simulink model "rre"  (Simulink 7.6)
settings: Solver=ode45  SolverMode=SingleTasking  StartTime=0  StopTime=10  FixedStep=0.002  RelTol=1e-3  AbsTol=1e-6
libraries: Solver_SF x1
settings Model: Creator=ywata  LastModifiedBy=bduprey  ExtModeTrigMode=oneshot  ExtModeArmWhenConnect=off
settings DataIOCC: LimitDataPoints=off  SignalLoggingName=sigsOut
settings OptimizationCC: BlockReduction=off  BooleanDataType=off  ExpressionDepthLimit=128
settings DebuggingCC: SaveWithParameterizedLinksMsg=none  SignalResolutionControl=TryResolveAllWithWarning  SolverPrmCheckMsg=none  MultiTaskDSMMsg=warning  MultiTaskCondExecSysMsg=none  FcnCallInpInsideContextMsg=Enable All
settings HardwareCC: TargetUnknown=on
settings RTWCC: TemplateMakefile=grt_vc.tmf
settings CodeAppCC: CustomSymbolStrType=$N$R$M_T
settings GRTTargetCC: TargetFcnLib=ansi_tfl_tmw.mat  TargetFunctionLibrary=C89/C90 (ANSI)

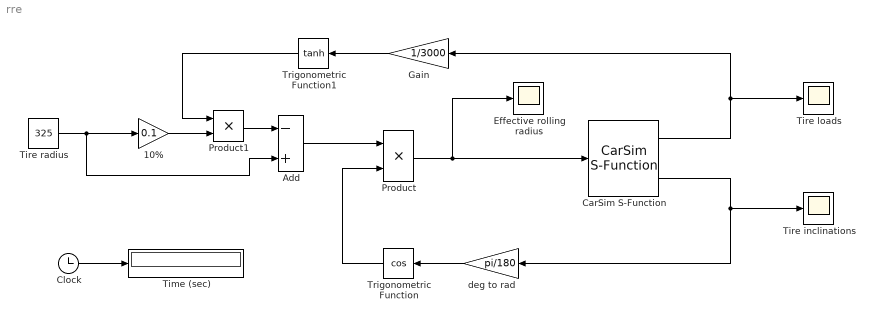
== system rre ==
  10% : Gain  Gain=0.1
  Add : Sum  Inputs=-+
  CarSim S-Function : Solver_SF/CarSim S-Function  Priority=1  SIMFILE=simfile.sim
  Clock : Clock
      settings: Decimation=10
  Effective rolling radius : Scope
      settings: TimeRange=6.3125  YMin=290  YMax=320  DataFormat=Array
  Gain : Gain  Gain=1/3000
  Product : Product
  Product1 : Product
  Time (sec) : Display
      settings: Format=bank  Decimation=100
  Tire inclinations : Scope
      settings: TimeRange=6.3125  YMin=-3  YMax=2  DataFormat=Array
  Tire loads : Scope
      settings: TimeRange=6.3125  YMin=0  YMax=6000  SaveName=ScopeData2  DataFormat=Array
  Tire radius : Constant  Value=325
  Trigonometric Function : Trigonometry  Operator=cos
  Trigonometric Function1 : Trigonometry  Operator=tanh
  deg to rad : Gain  Gain=pi/180
  wires:
  Clock/1 -> Time (sec)/1
  deg to rad/1 -> Trigonometric Function/1
  Product/1 -> CarSim S-Function/1, Effective rolling radius/1
  Trigonometric Function/1 -> Product/2
  CarSim S-Function/2 -> Tire inclinations/1, deg to rad/1
  Tire radius/1 -> Add/2, 10%/1
  10%/1 -> Product1/2
  CarSim S-Function/1 -> Gain/1, Tire loads/1
  Gain/1 -> Trigonometric Function1/1
  Trigonometric Function1/1 -> Product1/1
  Product1/1 -> Add/1
  Add/1 -> Product/1
